simulink model "mcb_resolver_host_read"  (R2026a)
settings: Solver=FixedStepDiscrete  StopTime=inf  EnableMultiTasking=on
InitFcn:
  | if( strcmp(get_param([gcs '/Serial Communication/HW_Selected'], 'Value'), '0'))
  |       set_param([gcs '/Host Serial Setup'], 'BaudRate', '12e6');
  | elseif( strcmp(get_param([gcs '/Serial Communication/HW_Selected'], 'Value'), '1'))
  |       set_param([gcs '/Host Serial Setup'], 'BaudRate', '5.625e6');
  | else
  | 
  | end
values from neighbouring files (symbols this model uses):
  dataType = 'single'    [mcb_resolver_f28379d_data.m]
  Ts_serial = Ts    (= 5e-05)    [mcb_resolver_f28379d_data.m]
libraries: instrumentseriallib x3
Description:
  | Host monitor for CN0276 AD2S1210 absolute resolver position in radians and degrees.
settings Model: Creator=The MathWorks, Inc.  LastModifiedBy=User
settings OptimizationCC: LifeSpan=1
settings HardwareCC: ProdHWDeviceType=32-bit Generic
settings RTWCC: SystemTargetFile=ert.tlc  GenerateReport=on  IncludeHyperlinkInReport=on  LaunchReport=on  GenerateTraceInfo=on  GenerateTraceReport=on  GenerateTraceReportSl=on  GenerateTraceReportSf=on  GenerateTraceReportEml=on  Description=Real-Time Workshop Embedded Coder
settings CodeAppCC: InternalIdentifier=Classic
settings ERTTargetCC: DynamicArrayContainerType=coder::array  MultiwordLength=2048.0  GenerateSampleERTMain=on

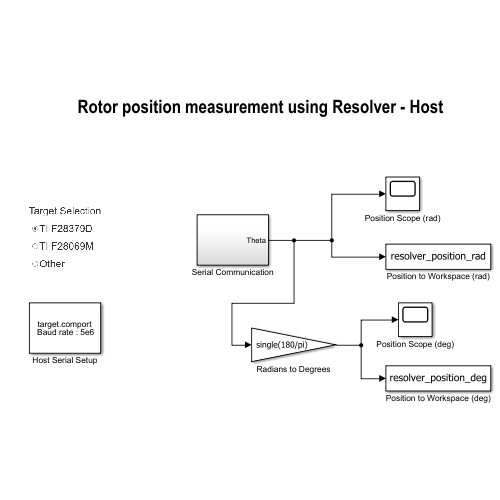
[thumbnail: Simulink's stored preview of the top-level diagram]
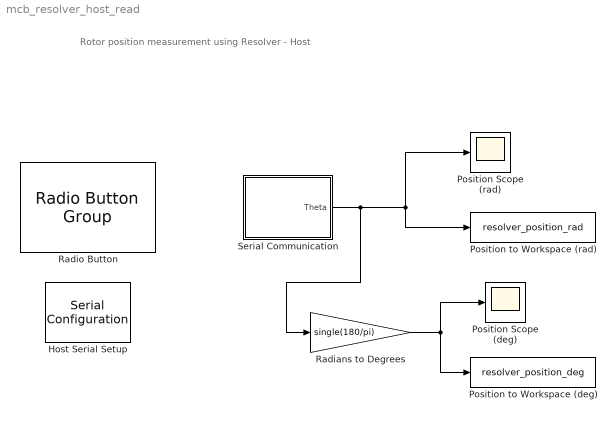
== system mcb_resolver_host_read ==
  note: Rotor position measurement using Resolver - Host
  Host Serial Setup : instrumentseriallib/Serial Configuration  Priority=-99  PortSel=target.comport  Port=target.comport  ComPort=target.comport  BaudRate=5e6  DataBits=8  Parity=none  StopBits=1  ByteOrder=little-endian  FlowControl=none  Timeout=2  SimulateUsing=Interpreted execution  BlockInModel=on  aMode=5
      settings: LibrarySourceBlock=mcblib/Protection and Diagnostics/Host Serial Setup
  Position Scope (deg) : Scope
      settings: TimeSpan=0.5  TimeUnits=Metric (based on Time Span)  ActiveDisplayYMinimum=-0.76150149106979348  ActiveDisplayYMaximum=6.8535134196281433  YLabel=Amplitude  DataLoggingMaxPoints=100
  Position Scope (rad) : Scope
      settings: TimeSpan=0.5  TimeUnits=Metric (based on Time Span)  ActiveDisplayYMinimum=-0.76150149106979348  ActiveDisplayYMaximum=6.8535134196281433  YLabel=Amplitude  DataLoggingMaxPoints=100
  Position to Workspace (deg) : ToWorkspace  VariableName=resolver_position_deg  SaveFormat=Structure With Time  SampleTime=-1
  Position to Workspace (rad) : ToWorkspace  VariableName=resolver_position_rad  SaveFormat=Structure With Time  SampleTime=-1
  Radians to Degrees : Gain  Gain=single(180/pi)  OutDataTypeStr=single
  Radio Button : RadioButtonGroup  LabelPosition=Hide  SelectedLabel=TI F28379D  ButtonGroupName=Target Selection
  Serial Communication : Subsystem
  wires:
  Serial Communication/1(Theta) -> Position Scope (rad)/1, Position to Workspace (rad)/1, Radians to Degrees/1
  Radians to Degrees/1 -> Position Scope (deg)/1, Position to Workspace (deg)/1

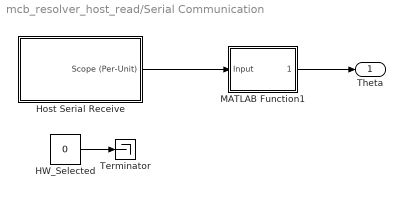
== system mcb_resolver_host_read/Serial Communication ==
  HW_Selected : Constant  Value=0  OutDataTypeStr=uint8
  Host Serial Receive : Subsystem  Variant=on
  MATLAB Function1 : MATLAB Function  TreatAsAtomicUnit=on
  Terminator : Terminator
  Theta : Outport
  wires:
  Host Serial Receive/1(Scope (Per-Unit)) -> MATLAB Function1/1(Input)
  HW_Selected/1 -> Terminator/1
  MATLAB Function1/1(Output1) -> Theta/1

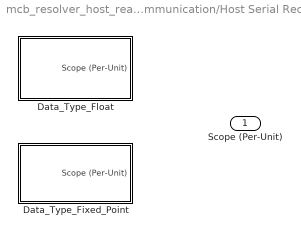
== system mcb_resolver_host_read/Serial Communication/Host Serial Receive ==
  Data_Type_Fixed_Point : Subsystem  VariantControl=~isequal(dataType, 'single')
  Data_Type_Float : Subsystem  VariantControl=isequal(dataType, 'single')
  Scope (Per-Unit) : Outport

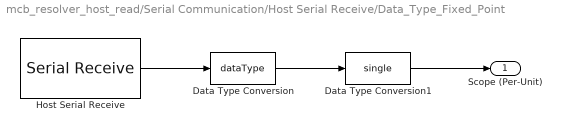
== system mcb_resolver_host_read/Serial Communication/Host Serial Receive/Data_Type_Fixed_Point ==
  Data Type Conversion : DataTypeConversion  OutDataTypeStr=dataType  ConvertRealWorld=Stored Integer (SI)  RndMeth=Simplest  SaturateOnIntegerOverflow=off
  Data Type Conversion1 : DataTypeConversion  OutDataTypeStr=single  RndMeth=Simplest  SaturateOnIntegerOverflow=off
  Host Serial Receive : instrumentseriallib/Serial Receive  PortSel=target.comport  Port=target.comport  ComPort=target.comport  DataType=uint32  SaveDataType=uint8  ToggleHeader=on  Header='SS'  ToggleDataSize=on  DataSize=[600 1]  ToggleTerminator=on  Terminator=Custom terminator  CustomTerminator='EE'  InputFormat=Row major  EnableBlockingMode=on  ActionDataUnavailable=Output custom value  ActionWhenDataUnavailable=Output custom value  CustomValue=4  SampleTime=600*Ts_serial  SimulateUsing=Interpreted execution  BlockInModel=on  aMode=5  LibraryInUse=instrumentlib
      settings: LibrarySourceBlock=mcblib/Protection and Diagnostics/Host Serial Receive
  Scope (Per-Unit) : Outport
  wires:
  Data Type Conversion/1 -> Data Type Conversion1/1
  Host Serial Receive/1 -> Data Type Conversion/1
  Data Type Conversion1/1 -> Scope (Per-Unit)/1

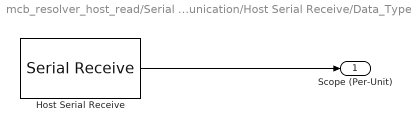
== system mcb_resolver_host_read/Serial Communication/Host Serial Receive/Data_Type_Float ==
  Host Serial Receive : instrumentseriallib/Serial Receive  PortSel=target.comport  Port=target.comport  ComPort=target.comport  DataType=single  SaveDataType=uint8  ToggleHeader=on  Header='SS'  ToggleDataSize=on  DataSize=[600 1]  ToggleTerminator=on  Terminator=Custom terminator  CustomTerminator='EE'  InputFormat=Row major  EnableBlockingMode=on  ActionDataUnavailable=Output custom value  ActionWhenDataUnavailable=Output custom value  CustomValue=4  SampleTime=600*Ts_serial  SimulateUsing=Interpreted execution  BlockInModel=on  aMode=5  LibraryInUse=instrumentlib
      settings: LibrarySourceBlock=mcblib/Protection and Diagnostics/Host Serial Receive
  Scope (Per-Unit) : Outport
  wires:
  Host Serial Receive/1 -> Scope (Per-Unit)/1

== matlab function mcb_resolver_host_read/Serial Communication/MATLAB Function1 ==
  data: Input input; Output1 output
function Output1  = unBuf(Input)
Output1 = Input(:, 1);
end
